simulink model "youbot_cinematique_BFpos14"  (R2014a)
settings: Solver=ode4  StartTime=0.0  StopTime=t(end)  FixedStep=Tech  RelTol=1e-3
values from neighbouring files (symbols this model uses):
  Tech = 1e-3    (= 0.001)    [script_youbot_Partie2.m]
  th_KUKA_1 = [0 -pi/2 -pi/3 +pi/2 0].'    [script_youbot_Partie2.m]
libraries: simulink x1
settings Model: CovSFcnEnable=on  Creator=Makarov_Mar  LastModifiedBy=Makarov_Mar
settings DebuggingCC: MergeDetectMultiDrivingBlocksExec=error  SolverPrmCheckMsg=none  FrameProcessingCompatibilityMsg=error

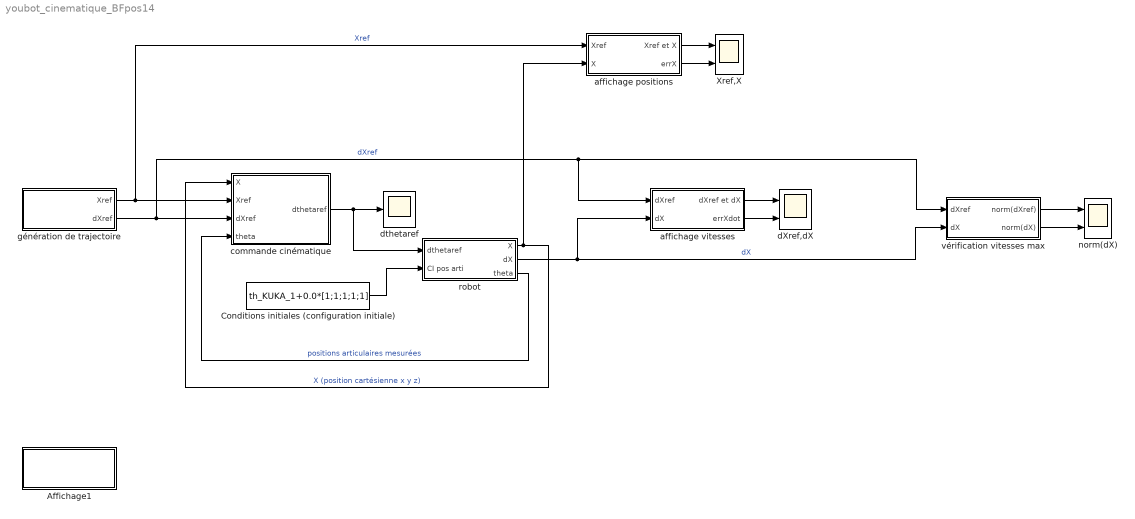
== system youbot_cinematique_BFpos14 ==
  Affichage1 : Subsystem  StopFcn=|
      | tps_sim =  pos_end.time;
      | PendX = pos_end.signals.values(:,1);
      | PendY = pos_end.signals.values(:,2);
      | PendZ = pos_end.signals.values(:,3);
      | 
      | figure(20)
      | plot3(Pt(1,:),Pt(2,:),Pt(3,:),'r','linewidth',2); hold on   
      | for k = 1:100:length(Pt)
      |   figure(20)
      |   plot3(0,0,0,'r.','markersize',20); grid on; hold on
      |   axis([-0.7 0.7 -0.7 0.7 0 +1])
      |   plot3(PendX(k),PendY(k),PendZ(k),'g.','markersize',20)
      |   xlabel('xB'); ylabel('yB'); zlabel('zB')
      |   title('xend : vert, yend : cyan, zend : rouge') 
      |   pause(0.1)
      | end
  Conditions initiales (configuration initiale) : Constant  Value=th_KUKA_1+0.0*[1;1;1;1;1]
  Xref,X : Scope  NumInputPorts=2
      settings: ShowLegends=on  YMin=-5~-5  YMax=5~5  SaveName=ScopeData4
  affichage positions : Subsystem
  affichage vitesses : Subsystem
  commande cinématique : Subsystem
  dXref,dX : Scope  NumInputPorts=2
      settings: ShowLegends=on  YMin=-5~-5  YMax=5~5  SaveName=ScopeData5
  dthetaref : Scope
      settings: ShowLegends=on  SaveName=ScopeData6
  génération de trajectoire : Subsystem
  norm(dX) : Scope  NumInputPorts=2
      settings: ShowLegends=on  YMin=-5~-5  YMax=5~5  SaveName=ScopeData2
  robot : Subsystem
  vérification vitesses max : Subsystem
  wires:
  génération de trajectoire/2(dXref) -> commande cinématique/3(dXref), affichage vitesses/1(dXref), vérification vitesses max/1(dXref)  "dXref"
  robot/3(theta) -> commande cinématique/4(theta)  "positions articulaires mesurées"
  génération de trajectoire/1(Xref) -> affichage positions/1(Xref), commande cinématique/2(Xref)  "Xref"
  robot/1(X) -> affichage positions/2(X), commande cinématique/1(X)  "X (position cartésienne x y z)"
  Conditions initiales (configuration initiale)/1 -> robot/2(CI pos arti)
  commande cinématique/1(dthetaref) -> robot/1(dthetaref), dthetaref/1
  robot/2(dX) -> vérification vitesses max/2(dX), affichage vitesses/2(dX)  "dX"
  vérification vitesses max/2(norm(dX)) -> norm(dX)/2
  vérification vitesses max/1(norm(dXref)) -> norm(dX)/1
  affichage positions/2(errX) -> Xref,X/2
  affichage positions/1(Xref et X) -> Xref,X/1
  affichage vitesses/1(dXref et dX) -> dXref,dX/1
  affichage vitesses/2(errXdot) -> dXref,dX/2

== system youbot_cinematique_BFpos14/Affichage1 ==

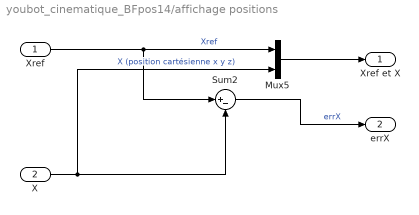
== system youbot_cinematique_BFpos14/affichage positions ==
  Xref : Inport
  X : Inport  Port=2
  Mux5 : Mux  Inputs=2
  Sum2 : Sum  Inputs=|+-
  Xref et X : Outport
  errX : Outport  Port=2
  wires:
  Xref/1 -> Sum2/1, Mux5/1  "Xref"
  Sum2/1 -> errX/1  "errX"
  X/1 -> Mux5/2, Sum2/2  "X (position cartésienne x y z)"
  Mux5/1 -> Xref et X/1

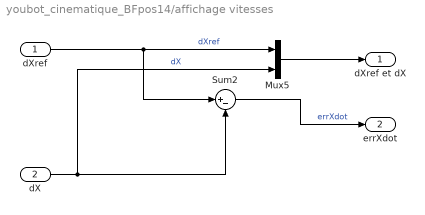
== system youbot_cinematique_BFpos14/affichage vitesses ==
  dXref : Inport
  dX : Inport  Port=2
  Mux5 : Mux  Inputs=2
  Sum2 : Sum  Inputs=|+-
  dXref et dX : Outport
  errXdot : Outport  Port=2
  wires:
  dXref/1 -> Sum2/1, Mux5/1  "dXref"
  Sum2/1 -> errXdot/1  "errXdot"
  dX/1 -> Mux5/2, Sum2/2  "dX"
  Mux5/1 -> dXref et dX/1

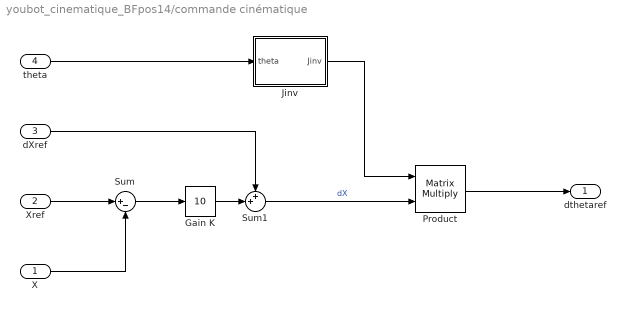
== system youbot_cinematique_BFpos14/commande cinématique ==
  X : Inport
  Xref : Inport  Port=2
  dXref : Inport  Port=3
  theta : Inport  Port=4  PortDimensions=5
  Gain K : simulink/Math Operations/Slider Gain  low=0  gain=10  high=100
  Jinv : MATLAB Function  TreatAsAtomicUnit=on
      settings: PermitHierarchicalResolution=ParametersOnly
  Product : Product  Multiplication=Matrix(*)
  Sum : Sum  Inputs=|+-
  Sum1 : Sum  Inputs=++|
  dthetaref : Outport
  wires:
  Jinv/1(Jinv) -> Product/1
  theta/1 -> Jinv/1(theta)
  Product/1 -> dthetaref/1
  Xref/1 -> Sum/1
  X/1 -> Sum/2
  Sum/1 -> Gain K/1
  Gain K/1 -> Sum1/2
  dXref/1 -> Sum1/1
  Sum1/1 -> Product/2  "dX"

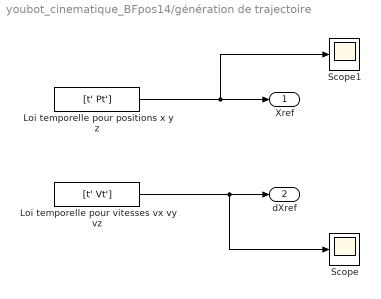
== system youbot_cinematique_BFpos14/génération de trajectoire ==
  Loi temporelle pour positions x y z : FromWorkspace  VariableName=[t' Pt']  SampleTime=Tech
  Loi temporelle pour vitesses vx vy vz : FromWorkspace  VariableName=[t' Vt']  SampleTime=Tech
  Scope : Scope
  Scope1 : Scope
  Xref : Outport
  dXref : Outport  Port=2
  wires:
  Loi temporelle pour positions x y z/1 -> Scope1/1, Xref/1
  Loi temporelle pour vitesses vx vy vz/1 -> Scope/1, dXref/1

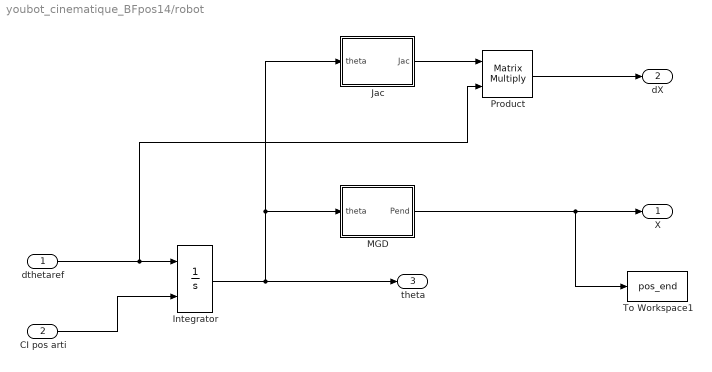
== system youbot_cinematique_BFpos14/robot ==
  dthetaref : Inport
  CI pos arti : Inport  Port=2
  Integrator : Integrator  InitialConditionSource=external
  Jac : MATLAB Function  TreatAsAtomicUnit=on
      settings: PermitHierarchicalResolution=ParametersOnly
  MGD : MATLAB Function  TreatAsAtomicUnit=on
      settings: PermitHierarchicalResolution=ParametersOnly
  Product : Product  Multiplication=Matrix(*)
  To Workspace1 : ToWorkspace  VariableName=pos_end  SaveFormat=Structure With Time  SampleTime=-1
  X : Outport
  dX : Outport  Port=2
  theta : Outport  Port=3
  wires:
  Jac/1(Jac) -> Product/1
  dthetaref/1 -> Product/2, Integrator/1
  Integrator/1 -> Jac/1(theta), MGD/1(theta), theta/1
  Product/1 -> dX/1
  CI pos arti/1 -> Integrator/2
  MGD/1(Pend) -> To Workspace1/1, X/1

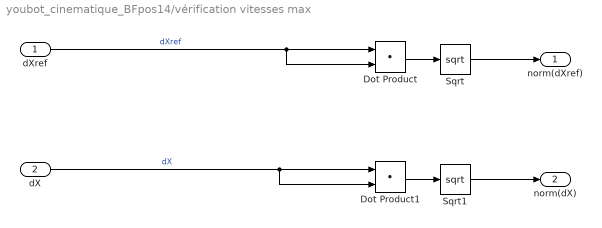
== system youbot_cinematique_BFpos14/vérification vitesses max ==
  dXref : Inport
  dX : Inport  Port=2
  Dot Product : DotProduct  InputSameDT=on  OutDataTypeStr=Inherit: Inherit via internal rule
  Dot Product1 : DotProduct  InputSameDT=on  OutDataTypeStr=Inherit: Inherit via internal rule
  Sqrt : Sqrt  SaturateOnIntegerOverflow=on
  Sqrt1 : Sqrt  SaturateOnIntegerOverflow=on
  norm(dXref) : Outport
  norm(dX) : Outport  Port=2
  wires:
  dXref/1 -> Dot Product/2, Dot Product/1  "dXref"
  Dot Product/1 -> Sqrt/1
  Sqrt/1 -> norm(dXref)/1
  dX/1 -> Dot Product1/2, Dot Product1/1  "dX"
  Dot Product1/1 -> Sqrt1/1
  Sqrt1/1 -> norm(dX)/1

== matlab function youbot_cinematique_BFpos14/commande cinématique/Jinv ==
  data: theta input; Jinv output
function Jinv = fcn(theta)
%#codegen

d2 = 0.033;
d3 = 0.155;
d4 = 0.135;
lend = 0.218;

th1 = theta(1);
th2 = theta(2);
th3 = theta(3);
th4 = theta(4);

Jac = Jacobian_youbot(d2,d3,d4,lend,th1,th2,th3,th4);

Jinv = pinv(Jac);

== matlab function youbot_cinematique_BFpos14/robot/Jac ==
  data: theta input; Jac output
function Jac = fcn(theta)
%#codegen

d2 = 0.033;
d3 = 0.155;
d4 = 0.135;
lend = 0.218;

th1 = theta(1);
th2 = theta(2);
th3 = theta(3);
th4 = theta(4);

Jac = Jacobian_youbot(d2,d3,d4,lend,th1,th2,th3,th4);

== matlab function youbot_cinematique_BFpos14/robot/MGD ==
  data: Pend output; theta input
function Pend = fcn(theta)
%#codegen

r1 = 0.147;
d2 = 0.033;
d3 = 0.155;
d4 = 0.135;
lend = 0.218;

th1 = theta(1);
th2 = theta(2);
th3 = theta(3);
th4 = theta(4);

Pend = MGD_end(d2,d3,d4,lend,r1,th1,th2,th3,th4);
